simulink model "SA_ACex4_ZADANIE3_1_MODEL"  (Simulink 9.1)
settings: Solver=VariableStepAuto  StartTime=0.0  StopTime=120  FixedStep=0.01  MaxStep=0.01  RelTol=1e-3  EnableMultiTasking=on
values from neighbouring files (symbols this model uses):
  omega_r = 0.25    [SA_ACex4_SKRYPT.m]
  sigma2e = 0.0    (= 0)    [SA_ACex4_SKRYPT.m]
  Ta = 0.005    [SA_ACex4_SKRYPT.m]
  Tc = 0.001    [SA_ACex4_SKRYPT.m]
  TF = 1.5*Ta    (= 0.0075)    [SA_ACex4_SKRYPT.m]
  Yr = 0.15    [SA_ACex4_SKRYPT.m]
libraries: simulink x1
settings Model: Creator=Gebruiker  LastModifiedBy=szymon
settings DataIOCC: LimitDataPoints=on  SignalLoggingSaveFormat=ModelDataLogs
settings OptimizationCC: InitFltsAndDblsToZero=on
settings DebuggingCC: SaveWithParameterizedLinksMsg=none  SignalResolutionControl=TryResolveAllWithWarning  SolverPrmCheckMsg=warning  MultiTaskDSMMsg=warning  MultiTaskCondExecSysMsg=none  FcnCallInpInsideContextMsg=warning
settings SFSimCC: SimUseLocalCustomCode=on
settings RTWCC: RTWUseLocalCustomCode=on
settings GRTTargetCC: TargetFcnLib=ansi_tfl_tmw.mat
settings ConfigComp: CovExternalEMLEnable=on

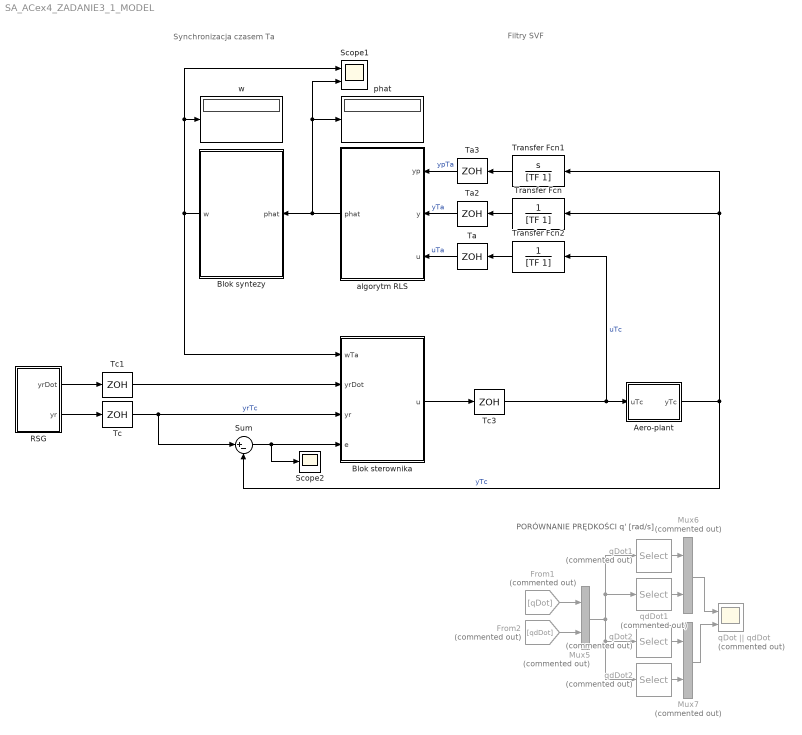
== system SA_ACex4_ZADANIE3_1_MODEL ==
  note: Synchronizacja czasem Ta
  note: Filtry SVF
  note: PORÓWNANIE PRĘDKOŚCI
      | q' [rad/s]
  Aero-plant : Subsystem
  Blok sterownika : Subsystem
  Blok syntezy : Subsystem
  From1 : From  Commented=on  GotoTag=qDot
  From2 : From  Commented=on  GotoTag=qdDot
  Mux5 : Mux  Commented=on  Inputs=2
  Mux6 : Mux  Commented=on  Inputs=2
  Mux7 : Mux  Commented=on  Inputs=2
  RSG : Subsystem
  Scope1 : Scope  NumInputPorts=2
  Scope2 : Scope
  Sum : Sum  Inputs=|+-
  Ta : ZeroOrderHold  SampleTime=Ta
  Ta2 : ZeroOrderHold  SampleTime=Ta
  Ta3 : ZeroOrderHold  SampleTime=Ta
  Tc : ZeroOrderHold  SampleTime=Tc
  Tc1 : ZeroOrderHold  SampleTime=Tc
  Tc3 : ZeroOrderHold  SampleTime=Tc
  Transfer Fcn : TransferFcn  Numerator=[0 1]  Denominator=[TF 1]
  Transfer Fcn1 : TransferFcn  Numerator=[1 0]  Denominator=[TF 1]
  Transfer Fcn2 : TransferFcn  Numerator=[0 1]  Denominator=[TF 1]
  algorytm RLS : Subsystem
  phat : Display
  qDot || qdDot : Scope  Commented=on  NumInputPorts=2
  qDot1 : Selector  Commented=on  InputPortWidth=4  IndexOptions=Index vector (dialog)  Indices=[1]  OutputSizes=1
  qDot2 : Selector  Commented=on  InputPortWidth=4  IndexOptions=Index vector (dialog)  Indices=[2]  OutputSizes=1
  qdDot1 : Selector  Commented=on  InputPortWidth=4  IndexOptions=Index vector (dialog)  Indices=[3]  OutputSizes=1
  qdDot2 : Selector  Commented=on  InputPortWidth=4  IndexOptions=Index vector (dialog)  Indices=[4]  OutputSizes=1
  w : Display
  wires:
  Aero-plant/1(yTc) -> Transfer Fcn1/1, Transfer Fcn/1, Sum/2  "yTc"
  RSG/1(yrDot) -> Tc1/1
  RSG/2(yr) -> Tc/1
  Tc/1 -> Sum/1, Blok sterownika/3(yr)  "yrTc"
  Tc3/1 -> Aero-plant/1(uTc), Transfer Fcn2/1  "uTc"
  Transfer Fcn1/1 -> Ta3/1
  Transfer Fcn2/1 -> Ta/1
  Transfer Fcn/1 -> Ta2/1
  Ta/1 -> algorytm RLS/3(u)  "uTa"
  Ta2/1 -> algorytm RLS/2(y)  "yTa"
  Ta3/1 -> algorytm RLS/1(yp)  "ypTa"
  Blok syntezy/1(w) -> Scope1/1, w/1, Blok sterownika/1(wTa)
  algorytm RLS/1(phat) -> phat/1, Scope1/2, Blok syntezy/1(phat)
  Tc1/1 -> Blok sterownika/2(yrDot)
  Sum/1 -> Scope2/1, Blok sterownika/4(e)
  Blok sterownika/1(u) -> Tc3/1
  Mux6/1 -> qDot || qdDot/1
  From2/1 -> Mux5/2
  Mux7/1 -> qDot || qdDot/2
  qdDot2/1 -> Mux7/2
  From1/1 -> Mux5/1
  qDot2/1 -> Mux7/1
  qDot1/1 -> Mux6/1
  Mux5/1 -> qdDot2/1, qDot2/1, qdDot1/1, qDot1/1
  qdDot1/1 -> Mux6/2

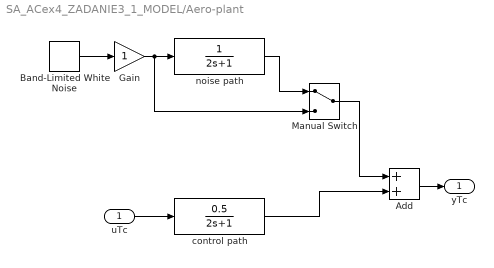
== system SA_ACex4_ZADANIE3_1_MODEL/Aero-plant ==
  uTc : Inport
  Add : Sum
  Band-Limited White Noise : simulink/Sources/Band-Limited White Noise  Cov=[sigma2e*Tc]  Ts=Tc  seed=[23341]
  Gain : Gain
  Manual Switch : ManualSwitch
  control path : TransferFcn  Numerator=[0.5]  Denominator=[2 1]
  noise path : TransferFcn  Denominator=[2 1]
  yTc : Outport
  wires:
  control path/1 -> Add/2
  Band-Limited White Noise/1 -> Gain/1
  Gain/1 -> Manual Switch/2, noise path/1
  Add/1 -> yTc/1
  uTc/1 -> control path/1
  noise path/1 -> Manual Switch/1
  Manual Switch/1 -> Add/1

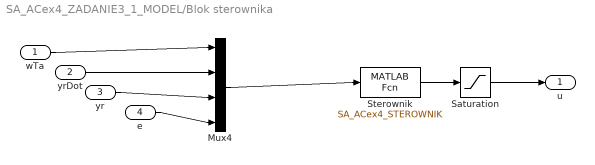
== system SA_ACex4_ZADANIE3_1_MODEL/Blok sterownika ==
  wTa : Inport
  yrDot : Inport  Port=2
  yr : Inport  Port=3
  e : Inport  Port=4
  Mux4 : Mux
  Saturation : Saturate  UpperLimit=pi/2  LowerLimit=-pi/2
  Sterownik : MATLABFcn  MATLABFcn=SA_ACex4_STEROWNIK  OutputDimensions=1
  u : Outport
  wires:
  Sterownik/1 -> Saturation/1
  Saturation/1 -> u/1
  Mux4/1 -> Sterownik/1
  e/1 -> Mux4/4
  yrDot/1 -> Mux4/2
  wTa/1 -> Mux4/1
  yr/1 -> Mux4/3

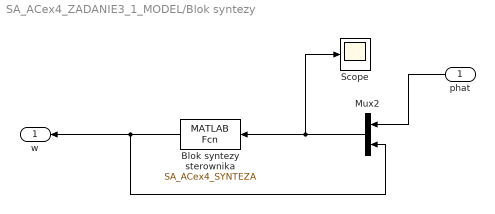
== system SA_ACex4_ZADANIE3_1_MODEL/Blok syntezy ==
  phat : Inport
  Blok syntezy sterownika : MATLABFcn  MATLABFcn=SA_ACex4_SYNTEZA
  Mux2 : Mux  Inputs=[2 3]
  Scope : Scope
  w : Outport
  wires:
  Mux2/1 -> Scope/1, Blok syntezy sterownika/1
  Blok syntezy sterownika/1 -> Mux2/2, w/1
  phat/1 -> Mux2/1

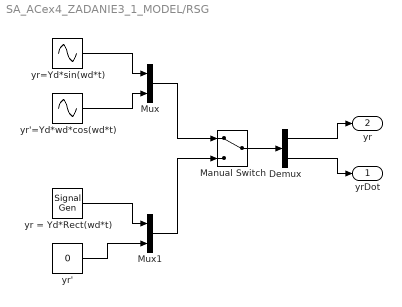
== system SA_ACex4_ZADANIE3_1_MODEL/RSG ==
  Demux : Demux  Outputs=2
  Manual Switch : ManualSwitch
  Mux : Mux  Inputs=2
  Mux1 : Mux  Inputs=2
  yr = Yd*Rect(wd*t) : SignalGenerator  WaveForm=square  Amplitude=Yr  Frequency=omega_r  Units=rad/sec
  yr' : Constant  Value=0
  yr'=Yd*wd*cos(wd*t) : Sin  Amplitude=Yr*omega_r  Frequency=omega_r  Phase=pi/2  SampleTime=0
  yr=Yd*sin(wd*t) : Sin  Amplitude=Yr  Frequency=omega_r  SampleTime=0
  yrDot : Outport
  yr : Outport  Port=2
  wires:
  yr=Yd*sin(wd*t)/1 -> Mux/1
  yr'=Yd*wd*cos(wd*t)/1 -> Mux/2
  yr = Yd*Rect(wd*t)/1 -> Mux1/1
  yr'/1 -> Mux1/2
  Mux/1 -> Manual Switch/1
  Mux1/1 -> Manual Switch/2
  Manual Switch/1 -> Demux/1
  Demux/1 -> yr/1
  Demux/2 -> yrDot/1

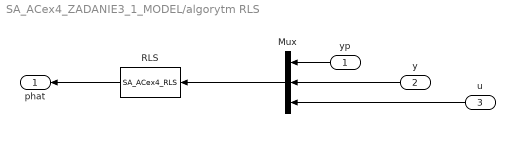
== system SA_ACex4_ZADANIE3_1_MODEL/algorytm RLS ==
  yp : Inport
  y : Inport  Port=2
  u : Inport  Port=3
  Mux : Mux  Inputs=3
  RLS : MATLABFcn  MATLABFcn=SA_ACex4_RLS  OutputDimensions=2
  phat : Outport
  wires:
  Mux/1 -> RLS/1
  RLS/1 -> phat/1
  u/1 -> Mux/3
  y/1 -> Mux/2
  yp/1 -> Mux/1
